simulink model "ex1_planar_robot_simulation_model"  (R2016b)
settings: Solver=FixedStepAuto  StartTime=0.0  StopTime=1  FixedStep=0.001  RelTol=1e-3  EnableMultiTasking=on
values from neighbouring files (symbols this model uses):
  a1 = u_gen(15)    [classical_joint_planar_robot_simulink.m]    (also in ct_gravit_planar_robot_simulink.m = u_gen(13); ct_pid_planar_robot_simulink.m; ct_planar_robot_simulink.m = u_gen(13); ex_planar_robot_2dof.m = 1)
  a2 = u_gen(16)    [classical_joint_planar_robot_simulink.m]    (also in ct_gravit_planar_robot_simulink.m = u_gen(14); ct_pid_planar_robot_simulink.m; ct_planar_robot_simulink.m = u_gen(14); ex_planar_robot_2dof.m = 1)
  b1 = u_gen(15)    [ct_gravit_planar_robot_simulink.m]    (also in ex_planar_robot_2dof.m = 0)
  b2 = u_gen(16)    [ct_gravit_planar_robot_simulink.m]    (also in ex_planar_robot_2dof.m = 0)
  g = u_gen(17)    [classical_joint_planar_robot_simulink.m]    (also in ct_gravit_planar_robot_simulink.m; ct_pid_planar_robot_simulink.m; ct_planar_robot_simulink.m = u_gen(15); ex_planar_robot_2dof.m = 9.81)
  m1 = u_gen(11)    [ac_controller_simulink.m]    (also in classical_joint_planar_robot_simulink.m = u_gen(13); ct_gravit_planar_robot_simulink.m; ct_pid_planar_robot_simulink.m = u_gen(13); ct_planar_robot_simulink.m)
  m2 = u_gen(12)    [ac_controller_simulink.m]    (also in classical_joint_planar_robot_simulink.m = u_gen(14); ct_gravit_planar_robot_simulink.m; ct_pid_planar_robot_simulink.m = u_gen(14); ct_planar_robot_simulink.m)
settings Model: Creator=sevimeda  LastModifiedBy=kargto
settings OptimizationCC: LifeSpan=inf
settings DebuggingCC: SFUnexpectedBacktrackingDiag=warning  SFNoUnconditionalDefaultTransitionDiag=warning  SFExecutionAtInitializationDiag=none
settings GRTTargetCC: TargetLangStandard=C89/C90 (ANSI)  GeneratePreprocessorConditionals=Disable all
settings ConfigComp: CovMetricSettings=dw  CovHtmlReporting=on  CovSaveCumulativeToWorkspaceVar=on  CovSaveSingleToWorkspaceVar=on  CovExternalEMLEnable=off

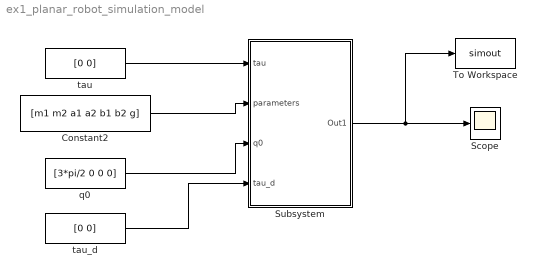
== system ex1_planar_robot_simulation_model ==
  Constant2 : Constant  Value=[m1 m2 a1 a2 b1 b2 g]
  Scope : Scope
  Subsystem : Subsystem
  To Workspace : ToWorkspace  VariableName=simout  SaveFormat=Structure With Time  SampleTime=-1
  q0 : Constant  Value=[3*pi/2 0 0 0]
  tau : Constant  Value=[0 0]
  tau_d : Constant  Value=[0 0]
  wires:
  Constant2/1 -> Subsystem/2(parameters)
  q0/1 -> Subsystem/3(q0)
  Subsystem/1(Out1) -> To Workspace/1, Scope/1
  tau/1 -> Subsystem/1(tau)
  tau_d/1 -> Subsystem/4(tau_d)

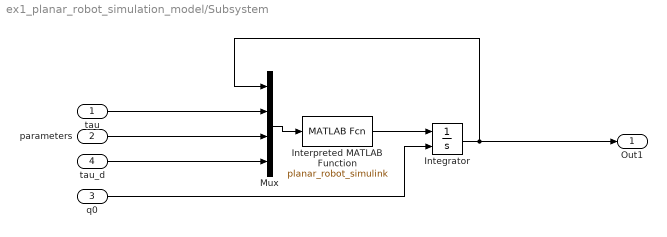
== system ex1_planar_robot_simulation_model/Subsystem ==
  tau : Inport
  parameters : Inport  Port=2
  q0 : Inport  Port=3
  tau_d : Inport  Port=4
  Integrator : Integrator  InitialConditionSource=external
  Interpreted MATLAB Function : MATLABFcn  MATLABFcn=planar_robot_simulink  OutputDimensions=4
  Mux : Mux
  Out1 : Outport
  wires:
  Interpreted MATLAB Function/1 -> Integrator/1
  q0/1 -> Integrator/2
  Mux/1 -> Interpreted MATLAB Function/1
  Integrator/1 -> Out1/1, Mux/1
  tau/1 -> Mux/2
  parameters/1 -> Mux/3
  tau_d/1 -> Mux/4
